simulink model "PLANET_v2"  (R2018b)
settings: Solver=FixedStepAuto  StartTime=0.0  StopTime=span-1  FixedStep=0.1  RelTol=1e-3
undefined symbols (not defined in the file): CHP_eta_el, CHP_eta_th, CHP_Pn, control, dh_demand, DH_elB_Cap, DH_elB_eff, DH_gas_B_Cap, DH_gas_B_eff, DH_HP_Cap, DH_HP_COP, DiscIntNeverNeededParam, dt, h_elD, lhd_demand, LHD_elB_Cap, LHD_elB_eff, LHD_gas_B_Cap, LHD_gas_B_eff, LHD_HP_Cap, LHD_HP_COP, Liion_cap, Liion_charge, Liion_dis, Liion_eff_ch, Liion_eff_dis, PCI, PtG_cap, PtG_eta_elcto, PtG_eta_meth, PtG_eta_th, PVPower, RES_curtailment_on_off, tt, WindPower
libraries: simulink x1
(part 4 of 5)

== system PLANET_v2/Control /Surplus dispacth/5: P2H P2G Li-ion /Li-ion control2/Free Battery MWh ==
  In1 : Inport
  Capacity [MWh] : Constant  Value=Capacity
  Product : Product
  Steate of Charge MAX [%] : Constant  Value=SoC_MAX/100
  Sum : Sum  Inputs=+|-
  Free space : Outport
  wires:
  Product/1 -> Sum/1
  Steate of Charge MAX [%]/1 -> Product/1
  Capacity [MWh]/1 -> Product/2
  Sum/1 -> Free space/1
  In1/1 -> Sum/2

== system PLANET_v2/Control /Surplus dispacth/5: P2H P2G Li-ion /Li-ion control2/If Action Subsystem ==
  Action Port : ActionPort  ActionType=then
  Constant : Constant  Value=0
  Bypassed surplus : Outport
  To battery : Outport  Port=2
  wires:
  Constant/1 -> To battery/1, Bypassed surplus/1

== system PLANET_v2/Control /Surplus dispacth/5: P2H P2G Li-ion /Li-ion control2/If Action Subsystem1 ==
  Surplus : Inport
  Action Port : ActionPort  ActionType=elseif
  Constant : Constant  Value=0
  Bypassed surplus : Outport
  To battery : Outport  Port=2
  wires:
  Surplus/1 -> To battery/1
  Constant/1 -> Bypassed surplus/1

== system PLANET_v2/Control /Surplus dispacth/5: P2H P2G Li-ion /Li-ion control2/If Action Subsystem2 ==
  Max charge : Inport
  Surplus : Inport  Port=2
  Action Port : ActionPort  ActionType=elseif
  Sum : Sum  Inputs=-+|
  Bypassed surplus : Outport
  To battery : Outport  Port=2
  wires:
  Max charge/1 -> Sum/1, To battery/1
  Sum/1 -> Bypassed surplus/1
  Surplus/1 -> Sum/2

== system PLANET_v2/Control /Surplus dispacth/5: P2H P2G Li-ion /Li-ion control2/If Action Subsystem4 ==
  free battery : Inport
  Surplus : Inport  Port=2
  Action Port : ActionPort  ActionType=else
  Sum : Sum  Inputs=-+|
  Bypassed surplus : Outport
  To battery : Outport  Port=2
  wires:
  free battery/1 -> To battery/1, Sum/1
  Sum/1 -> Bypassed surplus/1
  Surplus/1 -> Sum/2

== system PLANET_v2/Control /Surplus dispacth/5: P2H P2G Li-ion /Li-ion control2/MAX charge MW ==
  Charge capacity : Constant  Value=Max_charge
  Max battery charge : Outport
  wires:
  Charge capacity/1 -> Max battery charge/1

== system PLANET_v2/Control /Surplus dispacth/5: P2H P2G Li-ion /P2G control/If Action Subsystem ==
  Surplus : Inport
  Action Port : ActionPort  ActionType=else
  PtG capacity : Constant  Value=PtG_capacity
  Sum : Sum  Inputs=|+-
  New surplus : Outport
  wires:
  Sum/1 -> New surplus/1
  Surplus/1 -> Sum/1
  PtG capacity/1 -> Sum/2  "CH4 Power"

== system PLANET_v2/Control /Surplus dispacth/5: P2H P2G Li-ion /P2G control/If Action Subsystem1 ==
  Action Port : ActionPort  ActionType=elseif
  Constant : Constant  Value=0
  New surplus : Outport
  wires:
  Constant/1 -> New surplus/1

== system PLANET_v2/Control /Surplus dispacth/5: P2H P2G Li-ion /P2G control/If Action Subsystem2 ==
  Action Port : ActionPort  ActionType=then
  Constant : Constant  Value=0
  New surplus : Outport
  wires:
  Constant/1 -> New surplus/1

== system PLANET_v2/Control /Surplus dispacth/5: P2H P2G Li-ion /P2G control/Max P2G electric input ==
  P2G capacity : Constant  Value=PtG_capacity
  Max PtG input : Outport
  wires:
  P2G capacity/1 -> Max PtG input/1

== system PLANET_v2/Control /Surplus dispacth/5: P2H P2G Li-ion /P2H/Electric boiler DH ==
  Surplus : Inport
  th demand : Inport  Port=2
  If : If  NumInputs=2  IfExpression=u1 <= 0  ElseIfExpressions=u1 <= u2
  If Action Subsystem : Subsystem  TreatAsAtomicUnit=on
  If Action Subsystem1 : Subsystem  TreatAsAtomicUnit=on
  If Action Subsystem2 : Subsystem  TreatAsAtomicUnit=on
  Max el input : Constant  Value=Cap
  Max input control : Subsystem
  Merge : Merge  Inputs=3
  Merge1 : Merge  Inputs=3
  Sum1 : Sum  Inputs=|+-
  Sum2 : Sum  Inputs=++|
  th_eff : Gain  Gain=1/th_eff
  el cons : Outport
  New surplus : Outport  Port=2
  New th_d : Outport  Port=3
  wires:
  Surplus/1 -> Max input control/1(El input), Sum1/1
  th demand/1 -> If Action Subsystem1/2(Heat demand), If Action Subsystem2/2(Heat demand), th_eff/1, If Action Subsystem/2(Heat demand)
  Max input control/1(to PtH) -> If Action Subsystem/1(Surplus), If Action Subsystem1/1(Surplus), If/1, If Action Subsystem2/1(Surplus)
  Max el input/1 -> Max input control/2(Max el input)
  Max input control/2(Bypassed) -> Sum2/1
  Merge1/1 -> Sum2/2
  Sum2/1 -> Sum1/2, New surplus/1
  Sum1/1 -> el cons/1
  th_eff/1 -> If/2
  If Action Subsystem2/2(New heat demand) -> Merge/1
  Merge/1 -> New th_d/1
  If Action Subsystem1/2(New heat demand) -> Merge/2
  If/2 -> If Action Subsystem1/Action
  If Action Subsystem2/1(New surplus) -> Merge1/1
  If Action Subsystem/2(New heat demand) -> Merge/3
  If Action Subsystem/1(New surplus) -> Merge1/3
  If/3 -> If Action Subsystem/Action
  If/1 -> If Action Subsystem2/Action
  If Action Subsystem1/1(New surplus) -> Merge1/2

== system PLANET_v2/Control /Surplus dispacth/5: P2H P2G Li-ion /P2H/Electric boiler LHD ==
  Surplus : Inport
  th demand : Inport  Port=2
  If : If  NumInputs=2  IfExpression=u1 <= 0  ElseIfExpressions=u1 <= u2
  If Action Subsystem : Subsystem  TreatAsAtomicUnit=on
  If Action Subsystem1 : Subsystem  TreatAsAtomicUnit=on
  If Action Subsystem2 : Subsystem  TreatAsAtomicUnit=on
  Max el input : Constant  Value=Cap
  Max input control : Subsystem
  Merge : Merge  Inputs=3
  Merge1 : Merge  Inputs=3
  Sum1 : Sum  Inputs=|+-
  Sum2 : Sum  Inputs=++|
  th_eff : Gain  Gain=1/th_eff
  el cons : Outport
  New surplus : Outport  Port=2
  New th_d : Outport  Port=3
  wires:
  Surplus/1 -> Max input control/1(El input), Sum1/1
  th demand/1 -> If Action Subsystem1/2(Heat demand), If Action Subsystem2/2(Heat demand), th_eff/1, If Action Subsystem/2(Heat demand)
  Max input control/1(to PtH) -> If Action Subsystem/1(Surplus), If Action Subsystem1/1(Surplus), If/1, If Action Subsystem2/1(Surplus)
  Max el input/1 -> Max input control/2(Max el input)
  Max input control/2(Bypassed) -> Sum2/1
  Merge1/1 -> Sum2/2
  Sum2/1 -> Sum1/2, New surplus/1
  Sum1/1 -> el cons/1
  th_eff/1 -> If/2
  If Action Subsystem2/2(New heat demand) -> Merge/1
  Merge/1 -> New th_d/1
  If Action Subsystem1/2(New heat demand) -> Merge/2
  If/2 -> If Action Subsystem1/Action
  If Action Subsystem2/1(New surplus) -> Merge1/1
  If Action Subsystem/2(New heat demand) -> Merge/3
  If Action Subsystem/1(New surplus) -> Merge1/3
  If/3 -> If Action Subsystem/Action
  If/1 -> If Action Subsystem2/Action
  If Action Subsystem1/1(New surplus) -> Merge1/2

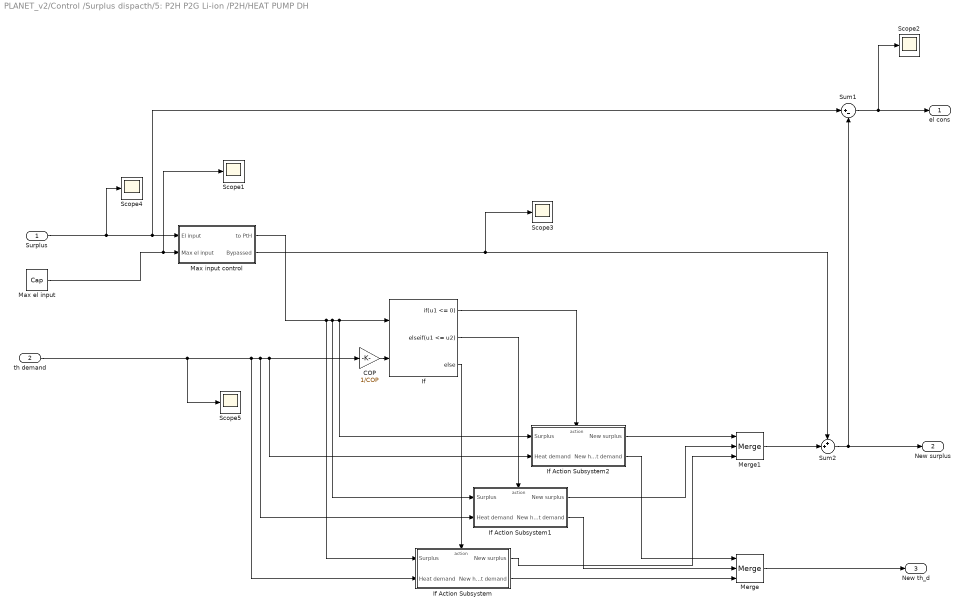
== system PLANET_v2/Control /Surplus dispacth/5: P2H P2G Li-ion /P2H/HEAT PUMP DH ==
  Surplus : Inport
  th demand : Inport  Port=2
  COP : Gain  Gain=1/COP
  If : If  NumInputs=2  IfExpression=u1 <= 0  ElseIfExpressions=u1 <= u2
  If Action Subsystem : Subsystem  TreatAsAtomicUnit=on
  If Action Subsystem1 : Subsystem  TreatAsAtomicUnit=on
  If Action Subsystem2 : Subsystem  TreatAsAtomicUnit=on
  Max el input : Constant  Value=Cap
  Max input control : Subsystem
  Merge : Merge  Inputs=3
  Merge1 : Merge  Inputs=3
  Scope{1..5} (5 alike) : Scope
  Sum1 : Sum  Inputs=|+-
  Sum2 : Sum  Inputs=++|
  el cons : Outport
  New surplus : Outport  Port=2
  New th_d : Outport  Port=3
  wires:
  Surplus/1 -> Max input control/1(El input), Sum1/1, Scope4/1
  th demand/1 -> If Action Subsystem1/2(Heat demand), If Action Subsystem2/2(Heat demand), COP/1, If Action Subsystem/2(Heat demand), Scope5/1
  Max input control/1(to PtH) -> If Action Subsystem/1(Surplus), If Action Subsystem1/1(Surplus), If/1, If Action Subsystem2/1(Surplus)
  Max el input/1 -> Scope1/1, Max input control/2(Max el input)
  Max input control/2(Bypassed) -> Sum2/1, Scope3/1
  Merge1/1 -> Sum2/2
  Sum2/1 -> Sum1/2, New surplus/1
  Sum1/1 -> el cons/1, Scope2/1
  COP/1 -> If/2
  If Action Subsystem2/2(New heat demand) -> Merge/1
  Merge/1 -> New th_d/1
  If Action Subsystem1/2(New heat demand) -> Merge/2
  If/2 -> If Action Subsystem1/Action
  If Action Subsystem2/1(New surplus) -> Merge1/1
  If Action Subsystem/2(New heat demand) -> Merge/3
  If Action Subsystem/1(New surplus) -> Merge1/3
  If/3 -> If Action Subsystem/Action
  If/1 -> If Action Subsystem2/Action
  If Action Subsystem1/1(New surplus) -> Merge1/2

== system PLANET_v2/Control /Surplus dispacth/5: P2H P2G Li-ion /P2H/HEAT PUMP local ==
  Surplus : Inport
  th demand : Inport  Port=2
  COP : Gain  Gain=1/COP
  If : If  NumInputs=2  IfExpression=u1 <= 0  ElseIfExpressions=u1 <= u2
  If Action Subsystem : Subsystem  TreatAsAtomicUnit=on
  If Action Subsystem1 : Subsystem  TreatAsAtomicUnit=on
  If Action Subsystem2 : Subsystem  TreatAsAtomicUnit=on
  Max el input : Constant  Value=Cap
  Max input control : Subsystem
  Merge : Merge  Inputs=3
  Merge1 : Merge  Inputs=3
  Sum1 : Sum  Inputs=|+-
  Sum2 : Sum  Inputs=++|
  el cons : Outport
  New surplus : Outport  Port=2
  New th_d : Outport  Port=3
  wires:
  Surplus/1 -> Max input control/1(El input), Sum1/1
  th demand/1 -> If Action Subsystem1/2(Heat demand), If Action Subsystem2/2(Heat demand), COP/1, If Action Subsystem/2(Heat demand)
  Max input control/1(to PtH) -> If Action Subsystem/1(Surplus), If Action Subsystem1/1(Surplus), If/1, If Action Subsystem2/1(Surplus)
  Max el input/1 -> Max input control/2(Max el input)
  Max input control/2(Bypassed) -> Sum2/1
  Merge1/1 -> Sum2/2
  Sum2/1 -> Sum1/2, New surplus/1
  Sum1/1 -> el cons/1
  COP/1 -> If/2
  If Action Subsystem2/2(New heat demand) -> Merge/1
  Merge/1 -> New th_d/1
  If Action Subsystem1/2(New heat demand) -> Merge/2
  If/2 -> If Action Subsystem1/Action
  If Action Subsystem2/1(New surplus) -> Merge1/1
  If Action Subsystem/2(New heat demand) -> Merge/3
  If Action Subsystem/1(New surplus) -> Merge1/3
  If/3 -> If Action Subsystem/Action
  If/1 -> If Action Subsystem2/Action
  If Action Subsystem1/1(New surplus) -> Merge1/2

== system PLANET_v2/Control /Surplus dispacth/0: Li-ion P2G P2H1/P2H/Electric boiler DH/If Action Subsystem ==
  Surplus : Inport
  Heat demand : Inport  Port=2
  Action Port : ActionPort  ActionType=else
  " " : Gain  Gain=1/th_eff
  Constant : Constant  Value=0
  Sum : Sum  Inputs=|+-
  New surplus : Outport
  New heat demand : Outport  Port=2
  wires:
  " "/1 -> Sum/2
  Sum/1 -> New surplus/1
  Heat demand/1 -> " "/1
  Surplus/1 -> Sum/1
  Constant/1 -> New heat demand/1

== system PLANET_v2/Control /Surplus dispacth/0: Li-ion P2G P2H1/P2H/Electric boiler DH/If Action Subsystem1 ==
  Surplus : Inport
  Heat demand : Inport  Port=2
  Action Port : ActionPort  ActionType=elseif
  Constant : Constant  Value=0
  Sum : Sum  Inputs=-+|
  th_eff : Gain  Gain=th_eff
  New surplus : Outport
  New heat demand : Outport  Port=2
  wires:
  Surplus/1 -> th_eff/1
  Constant/1 -> New surplus/1
  Sum/1 -> New heat demand/1
  th_eff/1 -> Sum/1
  Heat demand/1 -> Sum/2

== system PLANET_v2/Control /Surplus dispacth/0: Li-ion P2G P2H1/P2H/Electric boiler DH/If Action Subsystem2 ==
  Surplus : Inport
  Heat demand : Inport  Port=2
  Action Port : ActionPort  ActionType=then
  New surplus : Outport
  New heat demand : Outport  Port=2
  wires:
  Surplus/1 -> New surplus/1
  Heat demand/1 -> New heat demand/1

== system PLANET_v2/Control /Surplus dispacth/0: Li-ion P2G P2H1/P2H/Electric boiler DH/Max input control ==
  El input : Inport
  Max el input : Inport  Port=2
  If Action Subsystem3 : Subsystem  TreatAsAtomicUnit=on
  If Action Subsystem4 : Subsystem  TreatAsAtomicUnit=on
  If1 : If  NumInputs=2  IfExpression=u1 > u2
  Merge1 : Merge
  Merge2 : Merge
  to PtH : Outport
  Bypassed : Outport  Port=2
  wires:
  Merge2/1 -> to PtH/1
  If Action Subsystem3/1(to PtH) -> Merge2/1
  If Action Subsystem3/2(Bypassed surp) -> Merge1/1
  El input/1 -> If Action Subsystem4/1(Surplus), If Action Subsystem3/1(Surp), If1/1
  If1/1 -> If Action Subsystem3/Action
  If1/2 -> If Action Subsystem4/Action
  Max el input/1 -> If Action Subsystem3/2(Cap), If1/2
  If Action Subsystem4/1(to Pth) -> Merge2/2
  Merge1/1 -> Bypassed/1
  If Action Subsystem4/2(to Pth1) -> Merge1/2

== system PLANET_v2/Control /Surplus dispacth/0: Li-ion P2G P2H1/P2H/Electric boiler LHD/If Action Subsystem ==
  Surplus : Inport
  Heat demand : Inport  Port=2
  Action Port : ActionPort  ActionType=else
  " " : Gain  Gain=1/th_eff
  Constant : Constant  Value=0
  Sum : Sum  Inputs=|+-
  New surplus : Outport
  New heat demand : Outport  Port=2
  wires:
  " "/1 -> Sum/2
  Sum/1 -> New surplus/1
  Heat demand/1 -> " "/1
  Surplus/1 -> Sum/1
  Constant/1 -> New heat demand/1

== system PLANET_v2/Control /Surplus dispacth/0: Li-ion P2G P2H1/P2H/Electric boiler LHD/If Action Subsystem1 ==
  Surplus : Inport
  Heat demand : Inport  Port=2
  Action Port : ActionPort  ActionType=elseif
  Constant : Constant  Value=0
  Sum : Sum  Inputs=-+|
  th_eff : Gain  Gain=th_eff
  New surplus : Outport
  New heat demand : Outport  Port=2
  wires:
  Surplus/1 -> th_eff/1
  Constant/1 -> New surplus/1
  Sum/1 -> New heat demand/1
  th_eff/1 -> Sum/1
  Heat demand/1 -> Sum/2

== system PLANET_v2/Control /Surplus dispacth/0: Li-ion P2G P2H1/P2H/Electric boiler LHD/If Action Subsystem2 ==
  Surplus : Inport
  Heat demand : Inport  Port=2
  Action Port : ActionPort  ActionType=then
  New surplus : Outport
  New heat demand : Outport  Port=2
  wires:
  Surplus/1 -> New surplus/1
  Heat demand/1 -> New heat demand/1

== system PLANET_v2/Control /Surplus dispacth/0: Li-ion P2G P2H1/P2H/Electric boiler LHD/Max input control ==
  El input : Inport
  Max el input : Inport  Port=2
  If Action Subsystem3 : Subsystem  TreatAsAtomicUnit=on
  If Action Subsystem4 : Subsystem  TreatAsAtomicUnit=on
  If1 : If  NumInputs=2  IfExpression=u1 > u2
  Merge1 : Merge
  Merge2 : Merge
  to PtH : Outport
  Bypassed : Outport  Port=2
  wires:
  Merge2/1 -> to PtH/1
  If Action Subsystem3/1(to PtH) -> Merge2/1
  If Action Subsystem3/2(Bypassed surp) -> Merge1/1
  El input/1 -> If Action Subsystem4/1(Surplus), If Action Subsystem3/1(Surp), If1/1
  If1/1 -> If Action Subsystem3/Action
  If1/2 -> If Action Subsystem4/Action
  Max el input/1 -> If Action Subsystem3/2(Cap), If1/2
  If Action Subsystem4/1(to Pth) -> Merge2/2
  Merge1/1 -> Bypassed/1
  If Action Subsystem4/2(to Pth1) -> Merge1/2

== system PLANET_v2/Control /Surplus dispacth/0: Li-ion P2G P2H1/P2H/HEAT PUMP DH/If Action Subsystem ==
  Surplus : Inport
  Heat demand : Inport  Port=2
  Action Port : ActionPort  ActionType=else
  " " : Gain  Gain=1/COP
  Constant : Constant  Value=0
  Sum : Sum  Inputs=|+-
  New surplus : Outport
  New heat demand : Outport  Port=2
  wires:
  " "/1 -> Sum/2
  Sum/1 -> New surplus/1
  Heat demand/1 -> " "/1
  Surplus/1 -> Sum/1
  Constant/1 -> New heat demand/1

== system PLANET_v2/Control /Surplus dispacth/0: Li-ion P2G P2H1/P2H/HEAT PUMP DH/If Action Subsystem1 ==
  Surplus : Inport
  Heat demand : Inport  Port=2
  Action Port : ActionPort  ActionType=elseif
  COP : Gain  Gain=COP
  Constant : Constant  Value=0
  Sum : Sum  Inputs=-+|
  New surplus : Outport
  New heat demand : Outport  Port=2
  wires:
  Surplus/1 -> COP/1
  Constant/1 -> New surplus/1
  Sum/1 -> New heat demand/1
  COP/1 -> Sum/1
  Heat demand/1 -> Sum/2

== system PLANET_v2/Control /Surplus dispacth/0: Li-ion P2G P2H1/P2H/HEAT PUMP DH/If Action Subsystem2 ==
  Surplus : Inport
  Heat demand : Inport  Port=2
  Action Port : ActionPort  ActionType=then
  New surplus : Outport
  New heat demand : Outport  Port=2
  wires:
  Surplus/1 -> New surplus/1
  Heat demand/1 -> New heat demand/1

== system PLANET_v2/Control /Surplus dispacth/0: Li-ion P2G P2H1/P2H/HEAT PUMP DH/Max input control ==
  El input : Inport
  Max el input : Inport  Port=2
  If Action Subsystem3 : Subsystem  TreatAsAtomicUnit=on
  If Action Subsystem4 : Subsystem  TreatAsAtomicUnit=on
  If1 : If  NumInputs=2  IfExpression=u1 > u2
  Merge1 : Merge
  Merge2 : Merge
  to PtH : Outport
  Bypassed : Outport  Port=2
  wires:
  Merge2/1 -> to PtH/1
  If Action Subsystem3/1(to PtH) -> Merge2/1
  If Action Subsystem3/2(Bypassed surp) -> Merge1/1
  El input/1 -> If Action Subsystem4/1(Surplus), If Action Subsystem3/1(Surp), If1/1
  If1/1 -> If Action Subsystem3/Action
  If1/2 -> If Action Subsystem4/Action
  Max el input/1 -> If Action Subsystem3/2(Cap), If1/2
  If Action Subsystem4/1(to Pth) -> Merge2/2
  Merge1/1 -> Bypassed/1
  If Action Subsystem4/2(to Pth1) -> Merge1/2

== system PLANET_v2/Control /Surplus dispacth/0: Li-ion P2G P2H1/P2H/HEAT PUMP local/If Action Subsystem ==
  Surplus : Inport
  Heat demand : Inport  Port=2
  Action Port : ActionPort  ActionType=else
  " " : Gain  Gain=1/COP
  Constant : Constant  Value=0
  Sum : Sum  Inputs=|+-
  New surplus : Outport
  New heat demand : Outport  Port=2
  wires:
  Heat demand/1 -> " "/1
  Sum/1 -> New surplus/1
  Surplus/1 -> Sum/1
  Constant/1 -> New heat demand/1
  " "/1 -> Sum/2

== system PLANET_v2/Control /Surplus dispacth/0: Li-ion P2G P2H1/P2H/HEAT PUMP local/If Action Subsystem1 ==
  Surplus : Inport
  Heat demand : Inport  Port=2
  Action Port : ActionPort  ActionType=elseif
  COP : Gain  Gain=COP
  Constant : Constant  Value=0
  Sum : Sum  Inputs=-+|
  New surplus : Outport
  New heat demand : Outport  Port=2
  wires:
  Constant/1 -> New surplus/1
  Surplus/1 -> COP/1
  Heat demand/1 -> Sum/2
  Sum/1 -> New heat demand/1
  COP/1 -> Sum/1

== system PLANET_v2/Control /Surplus dispacth/0: Li-ion P2G P2H1/P2H/HEAT PUMP local/If Action Subsystem2 ==
  Surplus : Inport
  Heat demand : Inport  Port=2
  Action Port : ActionPort  ActionType=then
  New surplus : Outport
  New heat demand : Outport  Port=2
  wires:
  Surplus/1 -> New surplus/1
  Heat demand/1 -> New heat demand/1

== system PLANET_v2/Control /Surplus dispacth/0: Li-ion P2G P2H1/P2H/HEAT PUMP local/Max input control ==
  El input : Inport
  Max el input : Inport  Port=2
  If Action Subsystem3 : Subsystem  TreatAsAtomicUnit=on
  If Action Subsystem4 : Subsystem  TreatAsAtomicUnit=on
  If1 : If  NumInputs=2  IfExpression=u1 > u2
  Merge1 : Merge
  Merge2 : Merge
  to PtH : Outport
  Bypassed : Outport  Port=2
  wires:
  Merge2/1 -> to PtH/1
  If Action Subsystem3/1(to PtH) -> Merge2/1
  If Action Subsystem3/2(Bypassed surp) -> Merge1/1
  El input/1 -> If Action Subsystem4/1(Surplus), If Action Subsystem3/1(Surp), If1/1
  If1/1 -> If Action Subsystem3/Action
  If1/2 -> If Action Subsystem4/Action
  Max el input/1 -> If Action Subsystem3/2(Cap), If1/2
  If Action Subsystem4/1(to Pth) -> Merge2/2
  Merge1/1 -> Bypassed/1
  If Action Subsystem4/2(to Pth1) -> Merge1/2

== system PLANET_v2/Control /Surplus dispacth/1: Li-ion P2H P2G/P2H/Electric boiler DH/If Action Subsystem ==
  Surplus : Inport
  Heat demand : Inport  Port=2
  Action Port : ActionPort  ActionType=else
  " " : Gain  Gain=1/th_eff
  Constant : Constant  Value=0
  Sum : Sum  Inputs=|+-
  New surplus : Outport
  New heat demand : Outport  Port=2
  wires:
  Constant/1 -> New heat demand/1
  Surplus/1 -> Sum/1
  Heat demand/1 -> " "/1
  Sum/1 -> New surplus/1
  " "/1 -> Sum/2

== system PLANET_v2/Control /Surplus dispacth/1: Li-ion P2H P2G/P2H/Electric boiler DH/If Action Subsystem1 ==
  Surplus : Inport
  Heat demand : Inport  Port=2
  Action Port : ActionPort  ActionType=elseif
  Constant : Constant  Value=0
  Sum : Sum  Inputs=-+|
  th_eff : Gain  Gain=th_eff
  New surplus : Outport
  New heat demand : Outport  Port=2
  wires:
  Heat demand/1 -> Sum/2
  th_eff/1 -> Sum/1
  Sum/1 -> New heat demand/1
  Constant/1 -> New surplus/1
  Surplus/1 -> th_eff/1

== system PLANET_v2/Control /Surplus dispacth/1: Li-ion P2H P2G/P2H/Electric boiler DH/If Action Subsystem2 ==
  Surplus : Inport
  Heat demand : Inport  Port=2
  Action Port : ActionPort  ActionType=then
  New surplus : Outport
  New heat demand : Outport  Port=2
  wires:
  Heat demand/1 -> New heat demand/1
  Surplus/1 -> New surplus/1

== system PLANET_v2/Control /Surplus dispacth/1: Li-ion P2H P2G/P2H/Electric boiler DH/Max input control ==
  El input : Inport
  Max el input : Inport  Port=2
  If Action Subsystem3 : Subsystem  TreatAsAtomicUnit=on
  If Action Subsystem4 : Subsystem  TreatAsAtomicUnit=on
  If1 : If  NumInputs=2  IfExpression=u1 > u2
  Merge1 : Merge
  Merge2 : Merge
  to PtH : Outport
  Bypassed : Outport  Port=2
  wires:
  If Action Subsystem4/2(to Pth1) -> Merge1/2
  Merge1/1 -> Bypassed/1
  If Action Subsystem4/1(to Pth) -> Merge2/2
  Max el input/1 -> If1/2, If Action Subsystem3/2(Cap)
  If1/2 -> If Action Subsystem4/Action
  If1/1 -> If Action Subsystem3/Action
  El input/1 -> If1/1, If Action Subsystem3/1(Surp), If Action Subsystem4/1(Surplus)
  If Action Subsystem3/2(Bypassed surp) -> Merge1/1
  If Action Subsystem3/1(to PtH) -> Merge2/1
  Merge2/1 -> to PtH/1

== system PLANET_v2/Control /Surplus dispacth/1: Li-ion P2H P2G/P2H/Electric boiler LHD/If Action Subsystem ==
  Surplus : Inport
  Heat demand : Inport  Port=2
  Action Port : ActionPort  ActionType=else
  " " : Gain  Gain=1/th_eff
  Constant : Constant  Value=0
  Sum : Sum  Inputs=|+-
  New surplus : Outport
  New heat demand : Outport  Port=2
  wires:
  Constant/1 -> New heat demand/1
  Surplus/1 -> Sum/1
  Heat demand/1 -> " "/1
  Sum/1 -> New surplus/1
  " "/1 -> Sum/2

== system PLANET_v2/Control /Surplus dispacth/1: Li-ion P2H P2G/P2H/Electric boiler LHD/If Action Subsystem1 ==
  Surplus : Inport
  Heat demand : Inport  Port=2
  Action Port : ActionPort  ActionType=elseif
  Constant : Constant  Value=0
  Sum : Sum  Inputs=-+|
  th_eff : Gain  Gain=th_eff
  New surplus : Outport
  New heat demand : Outport  Port=2
  wires:
  Heat demand/1 -> Sum/2
  th_eff/1 -> Sum/1
  Sum/1 -> New heat demand/1
  Constant/1 -> New surplus/1
  Surplus/1 -> th_eff/1

== system PLANET_v2/Control /Surplus dispacth/1: Li-ion P2H P2G/P2H/Electric boiler LHD/If Action Subsystem2 ==
  Surplus : Inport
  Heat demand : Inport  Port=2
  Action Port : ActionPort  ActionType=then
  New surplus : Outport
  New heat demand : Outport  Port=2
  wires:
  Heat demand/1 -> New heat demand/1
  Surplus/1 -> New surplus/1

== system PLANET_v2/Control /Surplus dispacth/1: Li-ion P2H P2G/P2H/Electric boiler LHD/Max input control ==
  El input : Inport
  Max el input : Inport  Port=2
  If Action Subsystem3 : Subsystem  TreatAsAtomicUnit=on
  If Action Subsystem4 : Subsystem  TreatAsAtomicUnit=on
  If1 : If  NumInputs=2  IfExpression=u1 > u2
  Merge1 : Merge
  Merge2 : Merge
  to PtH : Outport
  Bypassed : Outport  Port=2
  wires:
  If Action Subsystem4/2(to Pth1) -> Merge1/2
  Merge1/1 -> Bypassed/1
  If Action Subsystem4/1(to Pth) -> Merge2/2
  Max el input/1 -> If1/2, If Action Subsystem3/2(Cap)
  If1/2 -> If Action Subsystem4/Action
  If1/1 -> If Action Subsystem3/Action
  El input/1 -> If1/1, If Action Subsystem3/1(Surp), If Action Subsystem4/1(Surplus)
  If Action Subsystem3/2(Bypassed surp) -> Merge1/1
  If Action Subsystem3/1(to PtH) -> Merge2/1
  Merge2/1 -> to PtH/1

== system PLANET_v2/Control /Surplus dispacth/1: Li-ion P2H P2G/P2H/HEAT PUMP DH/If Action Subsystem ==
  Surplus : Inport
  Heat demand : Inport  Port=2
  Action Port : ActionPort  ActionType=else
  " " : Gain  Gain=1/COP
  Constant : Constant  Value=0
  Sum : Sum  Inputs=|+-
  New surplus : Outport
  New heat demand : Outport  Port=2
  wires:
  Constant/1 -> New heat demand/1
  Surplus/1 -> Sum/1
  Heat demand/1 -> " "/1
  Sum/1 -> New surplus/1
  " "/1 -> Sum/2

== system PLANET_v2/Control /Surplus dispacth/1: Li-ion P2H P2G/P2H/HEAT PUMP DH/If Action Subsystem1 ==
  Surplus : Inport
  Heat demand : Inport  Port=2
  Action Port : ActionPort  ActionType=elseif
  COP : Gain  Gain=COP
  Constant : Constant  Value=0
  Sum : Sum  Inputs=-+|
  New surplus : Outport
  New heat demand : Outport  Port=2
  wires:
  Heat demand/1 -> Sum/2
  COP/1 -> Sum/1
  Sum/1 -> New heat demand/1
  Constant/1 -> New surplus/1
  Surplus/1 -> COP/1

== system PLANET_v2/Control /Surplus dispacth/1: Li-ion P2H P2G/P2H/HEAT PUMP DH/If Action Subsystem2 ==
  Surplus : Inport
  Heat demand : Inport  Port=2
  Action Port : ActionPort  ActionType=then
  New surplus : Outport
  New heat demand : Outport  Port=2
  wires:
  Heat demand/1 -> New heat demand/1
  Surplus/1 -> New surplus/1

== system PLANET_v2/Control /Surplus dispacth/1: Li-ion P2H P2G/P2H/HEAT PUMP DH/Max input control ==
  El input : Inport
  Max el input : Inport  Port=2
  If Action Subsystem3 : Subsystem  TreatAsAtomicUnit=on
  If Action Subsystem4 : Subsystem  TreatAsAtomicUnit=on
  If1 : If  NumInputs=2  IfExpression=u1 > u2
  Merge1 : Merge
  Merge2 : Merge
  to PtH : Outport
  Bypassed : Outport  Port=2
  wires:
  If Action Subsystem4/2(to Pth1) -> Merge1/2
  Merge1/1 -> Bypassed/1
  If Action Subsystem4/1(to Pth) -> Merge2/2
  Max el input/1 -> If1/2, If Action Subsystem3/2(Cap)
  If1/2 -> If Action Subsystem4/Action
  If1/1 -> If Action Subsystem3/Action
  El input/1 -> If1/1, If Action Subsystem3/1(Surp), If Action Subsystem4/1(Surplus)
  If Action Subsystem3/2(Bypassed surp) -> Merge1/1
  If Action Subsystem3/1(to PtH) -> Merge2/1
  Merge2/1 -> to PtH/1

== system PLANET_v2/Control /Surplus dispacth/1: Li-ion P2H P2G/P2H/HEAT PUMP local/If Action Subsystem ==
  Surplus : Inport
  Heat demand : Inport  Port=2
  Action Port : ActionPort  ActionType=else
  " " : Gain  Gain=1/COP
  Constant : Constant  Value=0
  Sum : Sum  Inputs=|+-
  New surplus : Outport
  New heat demand : Outport  Port=2
  wires:
  Constant/1 -> New heat demand/1
  Surplus/1 -> Sum/1
  Heat demand/1 -> " "/1
  Sum/1 -> New surplus/1
  " "/1 -> Sum/2

== system PLANET_v2/Control /Surplus dispacth/1: Li-ion P2H P2G/P2H/HEAT PUMP local/If Action Subsystem1 ==
  Surplus : Inport
  Heat demand : Inport  Port=2
  Action Port : ActionPort  ActionType=elseif
  COP : Gain  Gain=COP
  Constant : Constant  Value=0
  Sum : Sum  Inputs=-+|
  New surplus : Outport
  New heat demand : Outport  Port=2
  wires:
  Heat demand/1 -> Sum/2
  COP/1 -> Sum/1
  Sum/1 -> New heat demand/1
  Constant/1 -> New surplus/1
  Surplus/1 -> COP/1

== system PLANET_v2/Control /Surplus dispacth/1: Li-ion P2H P2G/P2H/HEAT PUMP local/If Action Subsystem2 ==
  Surplus : Inport
  Heat demand : Inport  Port=2
  Action Port : ActionPort  ActionType=then
  New surplus : Outport
  New heat demand : Outport  Port=2
  wires:
  Heat demand/1 -> New heat demand/1
  Surplus/1 -> New surplus/1

== system PLANET_v2/Control /Surplus dispacth/1: Li-ion P2H P2G/P2H/HEAT PUMP local/Max input control ==
  El input : Inport
  Max el input : Inport  Port=2
  If Action Subsystem3 : Subsystem  TreatAsAtomicUnit=on
  If Action Subsystem4 : Subsystem  TreatAsAtomicUnit=on
  If1 : If  NumInputs=2  IfExpression=u1 > u2
  Merge1 : Merge
  Merge2 : Merge
  to PtH : Outport
  Bypassed : Outport  Port=2
  wires:
  If Action Subsystem4/2(to Pth1) -> Merge1/2
  Merge1/1 -> Bypassed/1
  If Action Subsystem4/1(to Pth) -> Merge2/2
  Max el input/1 -> If1/2, If Action Subsystem3/2(Cap)
  If1/2 -> If Action Subsystem4/Action
  If1/1 -> If Action Subsystem3/Action
  El input/1 -> If1/1, If Action Subsystem3/1(Surp), If Action Subsystem4/1(Surplus)
  If Action Subsystem3/2(Bypassed surp) -> Merge1/1
  If Action Subsystem3/1(to PtH) -> Merge2/1
  Merge2/1 -> to PtH/1

== system PLANET_v2/Control /Surplus dispacth/2: P2G Li-ion P2H/P2H/Electric boiler DH/If Action Subsystem ==
  Surplus : Inport
  Heat demand : Inport  Port=2
  Action Port : ActionPort  ActionType=else
  " " : Gain  Gain=1/th_eff
  Constant : Constant  Value=0
  Sum : Sum  Inputs=|+-
  New surplus : Outport
  New heat demand : Outport  Port=2
  wires:
  Constant/1 -> New heat demand/1
  Surplus/1 -> Sum/1
  Heat demand/1 -> " "/1
  Sum/1 -> New surplus/1
  " "/1 -> Sum/2

== system PLANET_v2/Control /Surplus dispacth/2: P2G Li-ion P2H/P2H/Electric boiler DH/If Action Subsystem1 ==
  Surplus : Inport
  Heat demand : Inport  Port=2
  Action Port : ActionPort  ActionType=elseif
  Constant : Constant  Value=0
  Sum : Sum  Inputs=-+|
  th_eff : Gain  Gain=th_eff
  New surplus : Outport
  New heat demand : Outport  Port=2
  wires:
  Heat demand/1 -> Sum/2
  th_eff/1 -> Sum/1
  Sum/1 -> New heat demand/1
  Constant/1 -> New surplus/1
  Surplus/1 -> th_eff/1

== system PLANET_v2/Control /Surplus dispacth/2: P2G Li-ion P2H/P2H/Electric boiler DH/If Action Subsystem2 ==
  Surplus : Inport
  Heat demand : Inport  Port=2
  Action Port : ActionPort  ActionType=then
  New surplus : Outport
  New heat demand : Outport  Port=2
  wires:
  Heat demand/1 -> New heat demand/1
  Surplus/1 -> New surplus/1

== system PLANET_v2/Control /Surplus dispacth/2: P2G Li-ion P2H/P2H/Electric boiler DH/Max input control ==
  El input : Inport
  Max el input : Inport  Port=2
  If Action Subsystem3 : Subsystem  TreatAsAtomicUnit=on
  If Action Subsystem4 : Subsystem  TreatAsAtomicUnit=on
  If1 : If  NumInputs=2  IfExpression=u1 > u2
  Merge1 : Merge
  Merge2 : Merge
  to PtH : Outport
  Bypassed : Outport  Port=2
  wires:
  If Action Subsystem4/2(to Pth1) -> Merge1/2
  Merge1/1 -> Bypassed/1
  If Action Subsystem4/1(to Pth) -> Merge2/2
  Max el input/1 -> If1/2, If Action Subsystem3/2(Cap)
  If1/2 -> If Action Subsystem4/Action
  If1/1 -> If Action Subsystem3/Action
  El input/1 -> If1/1, If Action Subsystem3/1(Surp), If Action Subsystem4/1(Surplus)
  If Action Subsystem3/2(Bypassed surp) -> Merge1/1
  If Action Subsystem3/1(to PtH) -> Merge2/1
  Merge2/1 -> to PtH/1

== system PLANET_v2/Control /Surplus dispacth/2: P2G Li-ion P2H/P2H/Electric boiler LHD/If Action Subsystem ==
  Surplus : Inport
  Heat demand : Inport  Port=2
  Action Port : ActionPort  ActionType=else
  " " : Gain  Gain=1/th_eff
  Constant : Constant  Value=0
  Sum : Sum  Inputs=|+-
  New surplus : Outport
  New heat demand : Outport  Port=2
  wires:
  Constant/1 -> New heat demand/1
  Surplus/1 -> Sum/1
  Heat demand/1 -> " "/1
  Sum/1 -> New surplus/1
  " "/1 -> Sum/2

== system PLANET_v2/Control /Surplus dispacth/2: P2G Li-ion P2H/P2H/Electric boiler LHD/If Action Subsystem1 ==
  Surplus : Inport
  Heat demand : Inport  Port=2
  Action Port : ActionPort  ActionType=elseif
  Constant : Constant  Value=0
  Sum : Sum  Inputs=-+|
  th_eff : Gain  Gain=th_eff
  New surplus : Outport
  New heat demand : Outport  Port=2
  wires:
  Heat demand/1 -> Sum/2
  th_eff/1 -> Sum/1
  Sum/1 -> New heat demand/1
  Constant/1 -> New surplus/1
  Surplus/1 -> th_eff/1

== system PLANET_v2/Control /Surplus dispacth/2: P2G Li-ion P2H/P2H/Electric boiler LHD/If Action Subsystem2 ==
  Surplus : Inport
  Heat demand : Inport  Port=2
  Action Port : ActionPort  ActionType=then
  New surplus : Outport
  New heat demand : Outport  Port=2
  wires:
  Heat demand/1 -> New heat demand/1
  Surplus/1 -> New surplus/1

== system PLANET_v2/Control /Surplus dispacth/2: P2G Li-ion P2H/P2H/Electric boiler LHD/Max input control ==
  El input : Inport
  Max el input : Inport  Port=2
  If Action Subsystem3 : Subsystem  TreatAsAtomicUnit=on
  If Action Subsystem4 : Subsystem  TreatAsAtomicUnit=on
  If1 : If  NumInputs=2  IfExpression=u1 > u2
  Merge1 : Merge
  Merge2 : Merge
  to PtH : Outport
  Bypassed : Outport  Port=2
  wires:
  If Action Subsystem4/2(to Pth1) -> Merge1/2
  Merge1/1 -> Bypassed/1
  If Action Subsystem4/1(to Pth) -> Merge2/2
  Max el input/1 -> If1/2, If Action Subsystem3/2(Cap)
  If1/2 -> If Action Subsystem4/Action
  If1/1 -> If Action Subsystem3/Action
  El input/1 -> If1/1, If Action Subsystem3/1(Surp), If Action Subsystem4/1(Surplus)
  If Action Subsystem3/2(Bypassed surp) -> Merge1/1
  If Action Subsystem3/1(to PtH) -> Merge2/1
  Merge2/1 -> to PtH/1

== system PLANET_v2/Control /Surplus dispacth/2: P2G Li-ion P2H/P2H/HEAT PUMP DH/If Action Subsystem ==
  Surplus : Inport
  Heat demand : Inport  Port=2
  Action Port : ActionPort  ActionType=else
  " " : Gain  Gain=1/COP
  Constant : Constant  Value=0
  Sum : Sum  Inputs=|+-
  New surplus : Outport
  New heat demand : Outport  Port=2
  wires:
  Constant/1 -> New heat demand/1
  Surplus/1 -> Sum/1
  Heat demand/1 -> " "/1
  Sum/1 -> New surplus/1
  " "/1 -> Sum/2

== system PLANET_v2/Control /Surplus dispacth/2: P2G Li-ion P2H/P2H/HEAT PUMP DH/If Action Subsystem1 ==
  Surplus : Inport
  Heat demand : Inport  Port=2
  Action Port : ActionPort  ActionType=elseif
  COP : Gain  Gain=COP
  Constant : Constant  Value=0
  Sum : Sum  Inputs=-+|
  New surplus : Outport
  New heat demand : Outport  Port=2
  wires:
  Heat demand/1 -> Sum/2
  COP/1 -> Sum/1
  Sum/1 -> New heat demand/1
  Constant/1 -> New surplus/1
  Surplus/1 -> COP/1

== system PLANET_v2/Control /Surplus dispacth/2: P2G Li-ion P2H/P2H/HEAT PUMP DH/If Action Subsystem2 ==
  Surplus : Inport
  Heat demand : Inport  Port=2
  Action Port : ActionPort  ActionType=then
  New surplus : Outport
  New heat demand : Outport  Port=2
  wires:
  Heat demand/1 -> New heat demand/1
  Surplus/1 -> New surplus/1

== system PLANET_v2/Control /Surplus dispacth/2: P2G Li-ion P2H/P2H/HEAT PUMP DH/Max input control ==
  El input : Inport
  Max el input : Inport  Port=2
  If Action Subsystem3 : Subsystem  TreatAsAtomicUnit=on
  If Action Subsystem4 : Subsystem  TreatAsAtomicUnit=on
  If1 : If  NumInputs=2  IfExpression=u1 > u2
  Merge1 : Merge
  Merge2 : Merge
  to PtH : Outport
  Bypassed : Outport  Port=2
  wires:
  If Action Subsystem4/2(to Pth1) -> Merge1/2
  Merge1/1 -> Bypassed/1
  If Action Subsystem4/1(to Pth) -> Merge2/2
  Max el input/1 -> If1/2, If Action Subsystem3/2(Cap)
  If1/2 -> If Action Subsystem4/Action
  If1/1 -> If Action Subsystem3/Action
  El input/1 -> If1/1, If Action Subsystem3/1(Surp), If Action Subsystem4/1(Surplus)
  If Action Subsystem3/2(Bypassed surp) -> Merge1/1
  If Action Subsystem3/1(to PtH) -> Merge2/1
  Merge2/1 -> to PtH/1

== system PLANET_v2/Control /Surplus dispacth/2: P2G Li-ion P2H/P2H/HEAT PUMP local/If Action Subsystem ==
  Surplus : Inport
  Heat demand : Inport  Port=2
  Action Port : ActionPort  ActionType=else
  " " : Gain  Gain=1/COP
  Constant : Constant  Value=0
  Sum : Sum  Inputs=|+-
  New surplus : Outport
  New heat demand : Outport  Port=2
  wires:
  Constant/1 -> New heat demand/1
  Surplus/1 -> Sum/1
  Heat demand/1 -> " "/1
  Sum/1 -> New surplus/1
  " "/1 -> Sum/2

== system PLANET_v2/Control /Surplus dispacth/2: P2G Li-ion P2H/P2H/HEAT PUMP local/If Action Subsystem1 ==
  Surplus : Inport
  Heat demand : Inport  Port=2
  Action Port : ActionPort  ActionType=elseif
  COP : Gain  Gain=COP
  Constant : Constant  Value=0
  Sum : Sum  Inputs=-+|
  New surplus : Outport
  New heat demand : Outport  Port=2
  wires:
  Heat demand/1 -> Sum/2
  COP/1 -> Sum/1
  Sum/1 -> New heat demand/1
  Constant/1 -> New surplus/1
  Surplus/1 -> COP/1

== system PLANET_v2/Control /Surplus dispacth/2: P2G Li-ion P2H/P2H/HEAT PUMP local/If Action Subsystem2 ==
  Surplus : Inport
  Heat demand : Inport  Port=2
  Action Port : ActionPort  ActionType=then
  New surplus : Outport
  New heat demand : Outport  Port=2
  wires:
  Heat demand/1 -> New heat demand/1
  Surplus/1 -> New surplus/1

== system PLANET_v2/Control /Surplus dispacth/2: P2G Li-ion P2H/P2H/HEAT PUMP local/Max input control ==
  El input : Inport
  Max el input : Inport  Port=2
  If Action Subsystem3 : Subsystem  TreatAsAtomicUnit=on
  If Action Subsystem4 : Subsystem  TreatAsAtomicUnit=on
  If1 : If  NumInputs=2  IfExpression=u1 > u2
  Merge1 : Merge
  Merge2 : Merge
  to PtH : Outport
  Bypassed : Outport  Port=2
  wires:
  If Action Subsystem4/2(to Pth1) -> Merge1/2
  Merge1/1 -> Bypassed/1
  If Action Subsystem4/1(to Pth) -> Merge2/2
  Max el input/1 -> If1/2, If Action Subsystem3/2(Cap)
  If1/2 -> If Action Subsystem4/Action
  If1/1 -> If Action Subsystem3/Action
  El input/1 -> If1/1, If Action Subsystem3/1(Surp), If Action Subsystem4/1(Surplus)
  If Action Subsystem3/2(Bypassed surp) -> Merge1/1
  If Action Subsystem3/1(to PtH) -> Merge2/1
  Merge2/1 -> to PtH/1

== system PLANET_v2/Control /Surplus dispacth/3: P2G P2H Li-ion/P2H/Electric boiler DH/If Action Subsystem ==
  Surplus : Inport
  Heat demand : Inport  Port=2
  Action Port : ActionPort  ActionType=else
  " " : Gain  Gain=1/th_eff
  Constant : Constant  Value=0
  Sum : Sum  Inputs=|+-
  New surplus : Outport
  New heat demand : Outport  Port=2
  wires:
  Constant/1 -> New heat demand/1
  Surplus/1 -> Sum/1
  Heat demand/1 -> " "/1
  Sum/1 -> New surplus/1
  " "/1 -> Sum/2

== system PLANET_v2/Control /Surplus dispacth/3: P2G P2H Li-ion/P2H/Electric boiler DH/If Action Subsystem1 ==
  Surplus : Inport
  Heat demand : Inport  Port=2
  Action Port : ActionPort  ActionType=elseif
  Constant : Constant  Value=0
  Sum : Sum  Inputs=-+|
  th_eff : Gain  Gain=th_eff
  New surplus : Outport
  New heat demand : Outport  Port=2
  wires:
  Heat demand/1 -> Sum/2
  th_eff/1 -> Sum/1
  Sum/1 -> New heat demand/1
  Constant/1 -> New surplus/1
  Surplus/1 -> th_eff/1

== system PLANET_v2/Control /Surplus dispacth/3: P2G P2H Li-ion/P2H/Electric boiler DH/If Action Subsystem2 ==
  Surplus : Inport
  Heat demand : Inport  Port=2
  Action Port : ActionPort  ActionType=then
  New surplus : Outport
  New heat demand : Outport  Port=2
  wires:
  Heat demand/1 -> New heat demand/1
  Surplus/1 -> New surplus/1

== system PLANET_v2/Control /Surplus dispacth/3: P2G P2H Li-ion/P2H/Electric boiler DH/Max input control ==
  El input : Inport
  Max el input : Inport  Port=2
  If Action Subsystem3 : Subsystem  TreatAsAtomicUnit=on
  If Action Subsystem4 : Subsystem  TreatAsAtomicUnit=on
  If1 : If  NumInputs=2  IfExpression=u1 > u2
  Merge1 : Merge
  Merge2 : Merge
  to PtH : Outport
  Bypassed : Outport  Port=2
  wires:
  If Action Subsystem4/2(to Pth1) -> Merge1/2
  Merge1/1 -> Bypassed/1
  If Action Subsystem4/1(to Pth) -> Merge2/2
  Max el input/1 -> If1/2, If Action Subsystem3/2(Cap)
  If1/2 -> If Action Subsystem4/Action
  If1/1 -> If Action Subsystem3/Action
  El input/1 -> If1/1, If Action Subsystem3/1(Surp), If Action Subsystem4/1(Surplus)
  If Action Subsystem3/2(Bypassed surp) -> Merge1/1
  If Action Subsystem3/1(to PtH) -> Merge2/1
  Merge2/1 -> to PtH/1

== system PLANET_v2/Control /Surplus dispacth/3: P2G P2H Li-ion/P2H/Electric boiler LHD/If Action Subsystem ==
  Surplus : Inport
  Heat demand : Inport  Port=2
  Action Port : ActionPort  ActionType=else
  " " : Gain  Gain=1/th_eff
  Constant : Constant  Value=0
  Sum : Sum  Inputs=|+-
  New surplus : Outport
  New heat demand : Outport  Port=2
  wires:
  Constant/1 -> New heat demand/1
  Surplus/1 -> Sum/1
  Heat demand/1 -> " "/1
  Sum/1 -> New surplus/1
  " "/1 -> Sum/2

== system PLANET_v2/Control /Surplus dispacth/3: P2G P2H Li-ion/P2H/Electric boiler LHD/If Action Subsystem1 ==
  Surplus : Inport
  Heat demand : Inport  Port=2
  Action Port : ActionPort  ActionType=elseif
  Constant : Constant  Value=0
  Sum : Sum  Inputs=-+|
  th_eff : Gain  Gain=th_eff
  New surplus : Outport
  New heat demand : Outport  Port=2
  wires:
  Heat demand/1 -> Sum/2
  th_eff/1 -> Sum/1
  Sum/1 -> New heat demand/1
  Constant/1 -> New surplus/1
  Surplus/1 -> th_eff/1

== system PLANET_v2/Control /Surplus dispacth/3: P2G P2H Li-ion/P2H/Electric boiler LHD/If Action Subsystem2 ==
  Surplus : Inport
  Heat demand : Inport  Port=2
  Action Port : ActionPort  ActionType=then
  New surplus : Outport
  New heat demand : Outport  Port=2
  wires:
  Heat demand/1 -> New heat demand/1
  Surplus/1 -> New surplus/1

== system PLANET_v2/Control /Surplus dispacth/3: P2G P2H Li-ion/P2H/Electric boiler LHD/Max input control ==
  El input : Inport
  Max el input : Inport  Port=2
  If Action Subsystem3 : Subsystem  TreatAsAtomicUnit=on
  If Action Subsystem4 : Subsystem  TreatAsAtomicUnit=on
  If1 : If  NumInputs=2  IfExpression=u1 > u2
  Merge1 : Merge
  Merge2 : Merge
  Scope : Scope  NumInputPorts=2
  Scope1 : Scope
  to PtH : Outport
  Bypassed : Outport  Port=2
  wires:
  If Action Subsystem4/2(to Pth1) -> Merge1/2
  Merge1/1 -> Bypassed/1, Scope1/1
  If Action Subsystem4/1(to Pth) -> Merge2/2
  Max el input/1 -> If1/2, If Action Subsystem3/2(Cap), Scope/2
  If1/2 -> If Action Subsystem4/Action
  If1/1 -> If Action Subsystem3/Action
  El input/1 -> If1/1, If Action Subsystem3/1(Surp), If Action Subsystem4/1(Surplus), Scope/1
  If Action Subsystem3/2(Bypassed surp) -> Merge1/1
  If Action Subsystem3/1(to PtH) -> Merge2/1
  Merge2/1 -> to PtH/1

== system PLANET_v2/Control /Surplus dispacth/3: P2G P2H Li-ion/P2H/HEAT PUMP DH/If Action Subsystem ==
  Surplus : Inport
  Heat demand : Inport  Port=2
  Action Port : ActionPort  ActionType=else
  " " : Gain  Gain=1/COP
  Constant : Constant  Value=0
  Sum : Sum  Inputs=|+-
  New surplus : Outport
  New heat demand : Outport  Port=2
  wires:
  Constant/1 -> New heat demand/1
  Surplus/1 -> Sum/1
  Heat demand/1 -> " "/1
  Sum/1 -> New surplus/1
  " "/1 -> Sum/2

== system PLANET_v2/Control /Surplus dispacth/3: P2G P2H Li-ion/P2H/HEAT PUMP DH/If Action Subsystem1 ==
  Surplus : Inport
  Heat demand : Inport  Port=2
  Action Port : ActionPort  ActionType=elseif
  COP : Gain  Gain=COP
  Constant : Constant  Value=0
  Sum : Sum  Inputs=-+|
  New surplus : Outport
  New heat demand : Outport  Port=2
  wires:
  Heat demand/1 -> Sum/2
  COP/1 -> Sum/1
  Sum/1 -> New heat demand/1
  Constant/1 -> New surplus/1
  Surplus/1 -> COP/1

== system PLANET_v2/Control /Surplus dispacth/3: P2G P2H Li-ion/P2H/HEAT PUMP DH/If Action Subsystem2 ==
  Surplus : Inport
  Heat demand : Inport  Port=2
  Action Port : ActionPort  ActionType=then
  New surplus : Outport
  New heat demand : Outport  Port=2
  wires:
  Heat demand/1 -> New heat demand/1
  Surplus/1 -> New surplus/1

== system PLANET_v2/Control /Surplus dispacth/3: P2G P2H Li-ion/P2H/HEAT PUMP DH/Max input control ==
  El input : Inport
  Max el input : Inport  Port=2
  If Action Subsystem3 : Subsystem  TreatAsAtomicUnit=on
  If Action Subsystem4 : Subsystem  TreatAsAtomicUnit=on
  If1 : If  NumInputs=2  IfExpression=u1 > u2
  Merge1 : Merge
  Merge2 : Merge
  to PtH : Outport
  Bypassed : Outport  Port=2
  wires:
  If Action Subsystem4/2(to Pth1) -> Merge1/2
  Merge1/1 -> Bypassed/1
  If Action Subsystem4/1(to Pth) -> Merge2/2
  Max el input/1 -> If1/2, If Action Subsystem3/2(Cap)
  If1/2 -> If Action Subsystem4/Action
  If1/1 -> If Action Subsystem3/Action
  El input/1 -> If1/1, If Action Subsystem3/1(Surp), If Action Subsystem4/1(Surplus)
  If Action Subsystem3/2(Bypassed surp) -> Merge1/1
  If Action Subsystem3/1(to PtH) -> Merge2/1
  Merge2/1 -> to PtH/1

== system PLANET_v2/Control /Surplus dispacth/3: P2G P2H Li-ion/P2H/HEAT PUMP local/If Action Subsystem ==
  Surplus : Inport
  Heat demand : Inport  Port=2
  Action Port : ActionPort  ActionType=else
  " " : Gain  Gain=1/COP
  Constant : Constant  Value=0
  Sum : Sum  Inputs=|+-
  New surplus : Outport
  New heat demand : Outport  Port=2
  wires:
  Constant/1 -> New heat demand/1
  Surplus/1 -> Sum/1
  Heat demand/1 -> " "/1
  Sum/1 -> New surplus/1
  " "/1 -> Sum/2

== system PLANET_v2/Control /Surplus dispacth/3: P2G P2H Li-ion/P2H/HEAT PUMP local/If Action Subsystem1 ==
  Surplus : Inport
  Heat demand : Inport  Port=2
  Action Port : ActionPort  ActionType=elseif
  COP : Gain  Gain=COP
  Constant : Constant  Value=0
  Sum : Sum  Inputs=-+|
  New surplus : Outport
  New heat demand : Outport  Port=2
  wires:
  Heat demand/1 -> Sum/2
  COP/1 -> Sum/1
  Sum/1 -> New heat demand/1
  Constant/1 -> New surplus/1
  Surplus/1 -> COP/1

== system PLANET_v2/Control /Surplus dispacth/3: P2G P2H Li-ion/P2H/HEAT PUMP local/If Action Subsystem2 ==
  Surplus : Inport
  Heat demand : Inport  Port=2
  Action Port : ActionPort  ActionType=then
  New surplus : Outport
  New heat demand : Outport  Port=2
  wires:
  Heat demand/1 -> New heat demand/1
  Surplus/1 -> New surplus/1

== system PLANET_v2/Control /Surplus dispacth/3: P2G P2H Li-ion/P2H/HEAT PUMP local/Max input control ==
  El input : Inport
  Max el input : Inport  Port=2
  If Action Subsystem3 : Subsystem  TreatAsAtomicUnit=on
  If Action Subsystem4 : Subsystem  TreatAsAtomicUnit=on
  If1 : If  NumInputs=2  IfExpression=u1 > u2
  Merge1 : Merge
  Merge2 : Merge
  to PtH : Outport
  Bypassed : Outport  Port=2
  wires:
  If Action Subsystem4/2(to Pth1) -> Merge1/2
  Merge1/1 -> Bypassed/1
  If Action Subsystem4/1(to Pth) -> Merge2/2
  Max el input/1 -> If1/2, If Action Subsystem3/2(Cap)
  If1/2 -> If Action Subsystem4/Action
  If1/1 -> If Action Subsystem3/Action
  El input/1 -> If1/1, If Action Subsystem3/1(Surp), If Action Subsystem4/1(Surplus)
  If Action Subsystem3/2(Bypassed surp) -> Merge1/1
  If Action Subsystem3/1(to PtH) -> Merge2/1
  Merge2/1 -> to PtH/1

== system PLANET_v2/Control /Surplus dispacth/4: P2H Li-ion P2G/P2H/Electric boiler DH/If Action Subsystem ==
  Surplus : Inport
  Heat demand : Inport  Port=2
  Action Port : ActionPort  ActionType=else
  " " : Gain  Gain=1/th_eff
  Constant : Constant  Value=0
  Sum : Sum  Inputs=|+-
  New surplus : Outport
  New heat demand : Outport  Port=2
  wires:
  Constant/1 -> New heat demand/1
  Surplus/1 -> Sum/1
  Heat demand/1 -> " "/1
  Sum/1 -> New surplus/1
  " "/1 -> Sum/2

== system PLANET_v2/Control /Surplus dispacth/4: P2H Li-ion P2G/P2H/Electric boiler DH/If Action Subsystem1 ==
  Surplus : Inport
  Heat demand : Inport  Port=2
  Action Port : ActionPort  ActionType=elseif
  Constant : Constant  Value=0
  Sum : Sum  Inputs=-+|
  th_eff : Gain  Gain=th_eff
  New surplus : Outport
  New heat demand : Outport  Port=2
  wires:
  Heat demand/1 -> Sum/2
  th_eff/1 -> Sum/1
  Sum/1 -> New heat demand/1
  Constant/1 -> New surplus/1
  Surplus/1 -> th_eff/1

== system PLANET_v2/Control /Surplus dispacth/4: P2H Li-ion P2G/P2H/Electric boiler DH/If Action Subsystem2 ==
  Surplus : Inport
  Heat demand : Inport  Port=2
  Action Port : ActionPort  ActionType=then
  New surplus : Outport
  New heat demand : Outport  Port=2
  wires:
  Heat demand/1 -> New heat demand/1
  Surplus/1 -> New surplus/1

== system PLANET_v2/Control /Surplus dispacth/4: P2H Li-ion P2G/P2H/Electric boiler DH/Max input control ==
  El input : Inport
  Max el input : Inport  Port=2
  If Action Subsystem3 : Subsystem  TreatAsAtomicUnit=on
  If Action Subsystem4 : Subsystem  TreatAsAtomicUnit=on
  If1 : If  NumInputs=2  IfExpression=u1 > u2
  Merge1 : Merge
  Merge2 : Merge
  to PtH : Outport
  Bypassed : Outport  Port=2
  wires:
  If Action Subsystem4/2(to Pth1) -> Merge1/2
  Merge1/1 -> Bypassed/1
  If Action Subsystem4/1(to Pth) -> Merge2/2
  Max el input/1 -> If1/2, If Action Subsystem3/2(Cap)
  If1/2 -> If Action Subsystem4/Action
  If1/1 -> If Action Subsystem3/Action
  El input/1 -> If1/1, If Action Subsystem3/1(Surp), If Action Subsystem4/1(Surplus)
  If Action Subsystem3/2(Bypassed surp) -> Merge1/1
  If Action Subsystem3/1(to PtH) -> Merge2/1
  Merge2/1 -> to PtH/1

== system PLANET_v2/Control /Surplus dispacth/4: P2H Li-ion P2G/P2H/Electric boiler LHD/If Action Subsystem ==
  Surplus : Inport
  Heat demand : Inport  Port=2
  Action Port : ActionPort  ActionType=else
  " " : Gain  Gain=1/th_eff
  Constant : Constant  Value=0
  Sum : Sum  Inputs=|+-
  New surplus : Outport
  New heat demand : Outport  Port=2
  wires:
  Constant/1 -> New heat demand/1
  Surplus/1 -> Sum/1
  Heat demand/1 -> " "/1
  Sum/1 -> New surplus/1
  " "/1 -> Sum/2

== system PLANET_v2/Control /Surplus dispacth/4: P2H Li-ion P2G/P2H/Electric boiler LHD/If Action Subsystem1 ==
  Surplus : Inport
  Heat demand : Inport  Port=2
  Action Port : ActionPort  ActionType=elseif
  Constant : Constant  Value=0
  Sum : Sum  Inputs=-+|
  th_eff : Gain  Gain=th_eff
  New surplus : Outport
  New heat demand : Outport  Port=2
  wires:
  Heat demand/1 -> Sum/2
  th_eff/1 -> Sum/1
  Sum/1 -> New heat demand/1
  Constant/1 -> New surplus/1
  Surplus/1 -> th_eff/1

== system PLANET_v2/Control /Surplus dispacth/4: P2H Li-ion P2G/P2H/Electric boiler LHD/If Action Subsystem2 ==
  Surplus : Inport
  Heat demand : Inport  Port=2
  Action Port : ActionPort  ActionType=then
  New surplus : Outport
  New heat demand : Outport  Port=2
  wires:
  Heat demand/1 -> New heat demand/1
  Surplus/1 -> New surplus/1

== system PLANET_v2/Control /Surplus dispacth/4: P2H Li-ion P2G/P2H/Electric boiler LHD/Max input control ==
  El input : Inport
  Max el input : Inport  Port=2
  If Action Subsystem3 : Subsystem  TreatAsAtomicUnit=on
  If Action Subsystem4 : Subsystem  TreatAsAtomicUnit=on
  If1 : If  NumInputs=2  IfExpression=u1 > u2
  Merge1 : Merge
  Merge2 : Merge
  to PtH : Outport
  Bypassed : Outport  Port=2
  wires:
  If Action Subsystem4/2(to Pth1) -> Merge1/2
  Merge1/1 -> Bypassed/1
  If Action Subsystem4/1(to Pth) -> Merge2/2
  Max el input/1 -> If1/2, If Action Subsystem3/2(Cap)
  If1/2 -> If Action Subsystem4/Action
  If1/1 -> If Action Subsystem3/Action
  El input/1 -> If1/1, If Action Subsystem3/1(Surp), If Action Subsystem4/1(Surplus)
  If Action Subsystem3/2(Bypassed surp) -> Merge1/1
  If Action Subsystem3/1(to PtH) -> Merge2/1
  Merge2/1 -> to PtH/1

== system PLANET_v2/Control /Surplus dispacth/4: P2H Li-ion P2G/P2H/HEAT PUMP DH/If Action Subsystem ==
  Surplus : Inport
  Heat demand : Inport  Port=2
  Action Port : ActionPort  ActionType=else
  " " : Gain  Gain=1/COP
  Constant : Constant  Value=0
  Sum : Sum  Inputs=|+-
  New surplus : Outport
  New heat demand : Outport  Port=2
  wires:
  Constant/1 -> New heat demand/1
  Surplus/1 -> Sum/1
  Heat demand/1 -> " "/1
  Sum/1 -> New surplus/1
  " "/1 -> Sum/2
